simulink model "FinalModelDesign"  (R2012b)
settings: Solver=ode45  StartTime=0.0  StopTime=5  RelTol=1e-3
settings Model: SimulationMode=accelerator  Creator=kyle  LastModifiedBy=kyle
settings DataIOCC: InspectSignalLogs=on
settings OptimizationCC: InlineParams=on  SimCompilerOptimization=On
settings DebuggingCC: MergeDetectMultiDrivingBlocksExec=warning
settings ModelReferenceCC: UpdateModelReferenceTargets=IfOutOfDate
settings SFSimCC: SFSimEcho=off

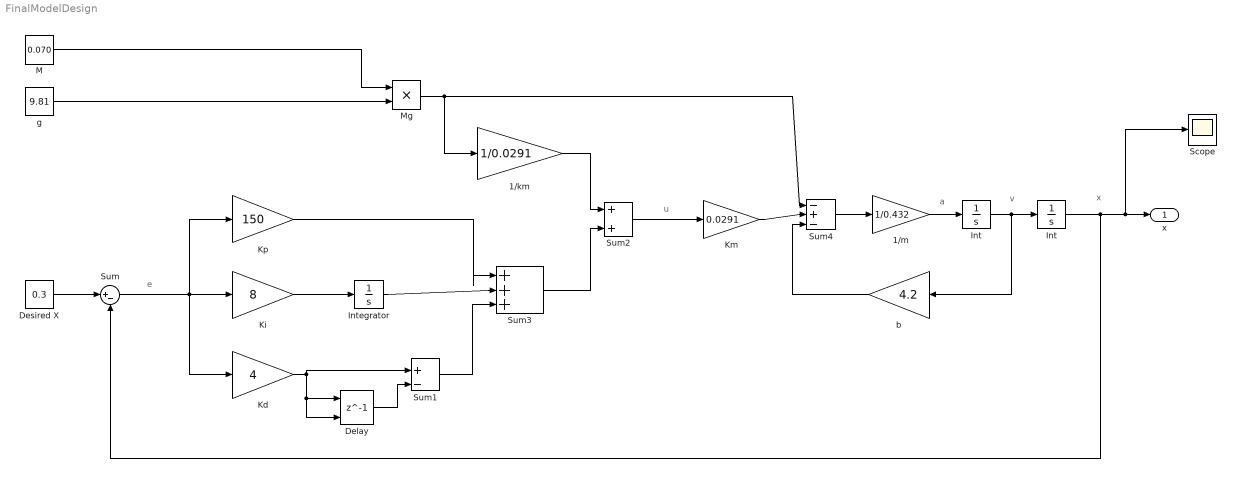
== system FinalModelDesign ==
  note: x
  note: u
  note: e
  note: a
  note: v
  1/km : Gain  Gain=1/0.0291
  1/m : Gain  Gain=1/0.432
  Delay : Delay  DelayLength=1  InitialConditionSource=Input port  InitialCondition=861  InputProcessing=Inherited  SampleTime=.01
      settings: InputPortMap=u0,p4
  Desired X : Constant  Value=0.3
  Int : Integrator
  "Int " : Integrator
  Integrator : Integrator
  Kd : Gain  Gain=4
  Ki : Gain  Gain=8
  Km : Gain  Gain=0.0291
  Kp : Gain  Gain=150
  M : Constant  Value=0.070
  Mg : Product  RndMeth=Zero
  Scope : Scope
  Sum : Sum  Inputs=|+-
  Sum1 : Sum  Inputs=|+-
  Sum2 : Sum  Inputs=|++
  Sum3 : Sum  Inputs=|+++
  Sum4 : Sum  Inputs=|-+-
  b : Gain  Gain=4.2
  g : Constant  Value=9.81
  x : Outport
  wires:
  Integrator/1 -> Sum3/2
  Ki/1 -> Integrator/1
  Kp/1 -> Sum3/1
  Sum1/1 -> Sum3/3
  Kd/1 -> Delay/2, Delay/1, Sum1/1
  Delay/1 -> Sum1/2
  Sum3/1 -> Sum2/2
  Sum/1 -> Kd/1, Kp/1, Ki/1
  g/1 -> Mg/2
  M/1 -> Mg/1
  1/km/1 -> Sum2/1
  Km/1 -> Sum4/2
  b/1 -> Sum4/3
  Sum4/1 -> 1/m/1
  "Int "/1 -> b/1, Int/1
  Mg/1 -> Sum4/1, 1/km/1
  1/m/1 -> "Int "/1
  Sum2/1 -> Km/1
  Desired X/1 -> Sum/1
  Int/1 -> Scope/1, x/1, Sum/2
